simulink model "test6_1_org"  (Simulink 10.0)
settings: Solver=ode45  StartTime=0.0  StopTime=10.0  RelTol=1e-3  EnableMultiTasking=on
libraries: commrandsrc2 x1, commnoisgen2 x1
settings Model: Creator=asus  LastModifiedBy=bhisma
settings DataIOCC: LimitDataPoints=on
settings DebuggingCC: UnderspecifiedInitializationDetection=Simplified  MergeDetectMultiDrivingBlocksExec=error  SolverPrmCheckMsg=warning
settings GRTTargetCC: GeneratePreprocessorConditionals=Disable all  CombineOutputUpdateFcns=on  GRTInterface=off
settings ConfigComp: CovExternalEMLEnable=off  CovSFcnEnable=off

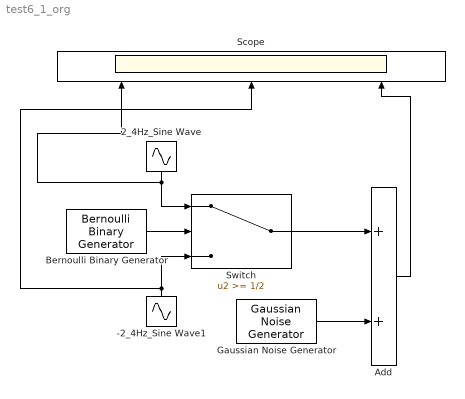
== system test6_1_org ==
  -2_4Hz_Sine Wave1 : Sin  Amplitude=-2  Frequency=pi  SampleTime=1/8000
  2_4Hz_Sine Wave : Sin  Amplitude=2  Frequency=pi  SampleTime=1/8000
  Add : Sum
  Bernoulli Binary Generator : commrandsrc2/Bernoulli Binary Generator  P=1  seed=61  Ts=1  frameBased=off  sampPerFrame=1  orient=off  outDataType=double
      settings: SourceProductName=Communications Toolbox  SourceProductBaseCode=CM
  Gaussian Noise Generator : commnoisgen2/Gaussian Noise Generator  m=0  d=1  s=41  Ts=1  frameBased=off  sampPerFrame=1  orient=off  outDataType=double
      settings: SourceProductName=Communications Toolbox  SourceProductBaseCode=CM
  Scope : Scope  NumInputPorts=3
  Switch : Switch  Threshold=1/2
  wires:
  Bernoulli Binary Generator/1 -> Switch/2
  2_4Hz_Sine Wave/1 -> Scope/1, Switch/1
  -2_4Hz_Sine Wave1/1 -> Scope/2, Switch/3
  Gaussian Noise Generator/1 -> Add/2
  Switch/1 -> Add/1
  Add/1 -> Scope/3
